simulink model "racing_modes_R2022a"  (R2022a)
settings: Solver=VariableStepAuto  StartTime=0.0  StopTime=10.0  RelTol=1e-3
settings Model: Creator=no  LastModifiedBy=no
settings ModelReferenceCC: EnableRefExpFcnMdlSchedulingChecks=off
settings RTWCC: Description=Generic Real-Time Target

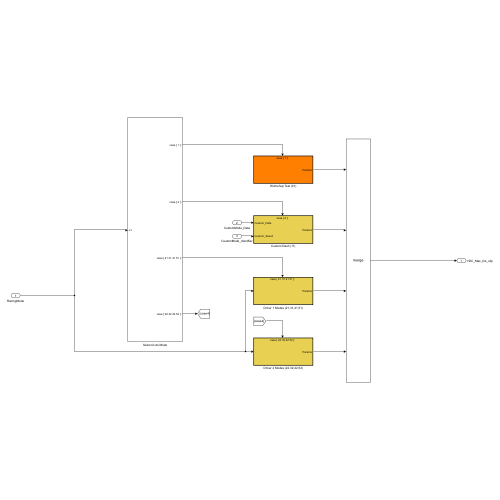
[thumbnail: Simulink's stored preview of the top-level diagram]
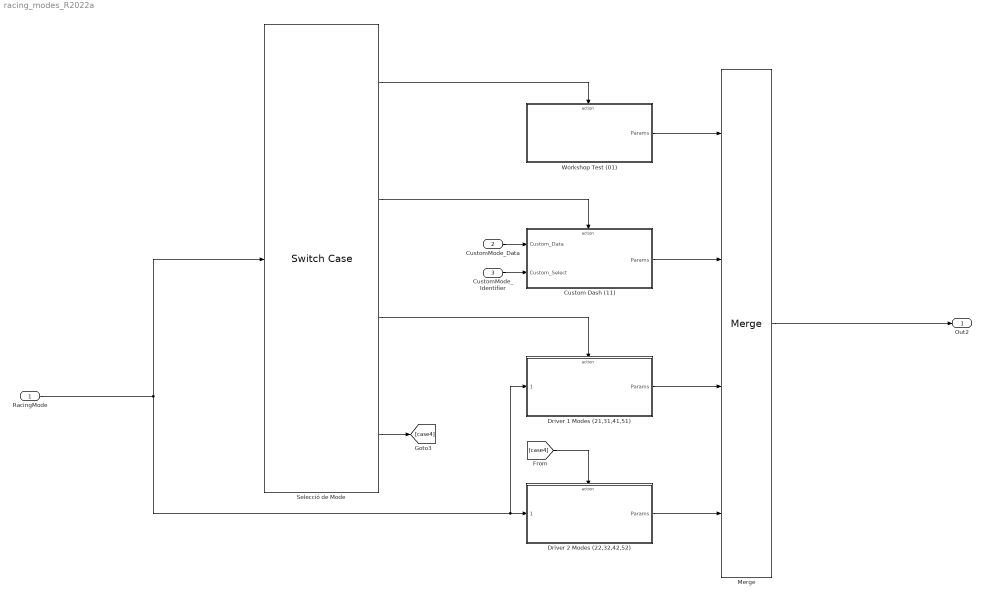
== system racing_modes_R2022a ==
  RacingMode : Inport  OutDataTypeStr=uint8
  CustomMode_Data : Inport  Port=2
  CustomMode_Identifier : Inport  Port=3
  Custom Dash (11) : Subsystem  TreatAsAtomicUnit=on
  Driver 1 Modes (21,31,41,51) : Subsystem  TreatAsAtomicUnit=on
  Driver 2 Modes (22,32,42,52) : Subsystem  TreatAsAtomicUnit=on
  Merge : Merge  Inputs=4
  Selecció de Mode : SwitchCase  CaseConditions={01, 2, [21,31,41,51], [22,32,42,52]}  ShowDefaultCase=off
  Workshop Test (01) : Subsystem  TreatAsAtomicUnit=on
  Out2 : Outport  SignalName=VDC_Max_tire_slip
  wires:
  CustomMode_Identifier/1 -> Custom Dash (11)/2(Custom_Select)
  Custom Dash (11)/1(Params) -> Merge/2
  RacingMode/1 -> Driver 1 Modes (21,31,41,51)/1(" "), Driver 2 Modes (22,32,42,52)/1(" "), Selecció de Mode/1
  Workshop Test (01)/1(Params) -> Merge/1
  CustomMode_Data/1 -> Custom Dash (11)/1(Custom_Data)
  Driver 1 Modes (21,31,41,51)/1(Params) -> Merge/3
  Driver 2 Modes (22,32,42,52)/1(Params) -> Merge/4
  Selecció de Mode/4 -> [case4]
  [case4] -> Driver 2 Modes (22,32,42,52)/Action
  Selecció de Mode/1 -> Workshop Test (01)/Action
  Selecció de Mode/2 -> Custom Dash (11)/Action
  Selecció de Mode/3 -> Driver 1 Modes (21,31,41,51)/Action
  Merge/1 -> Out2/1

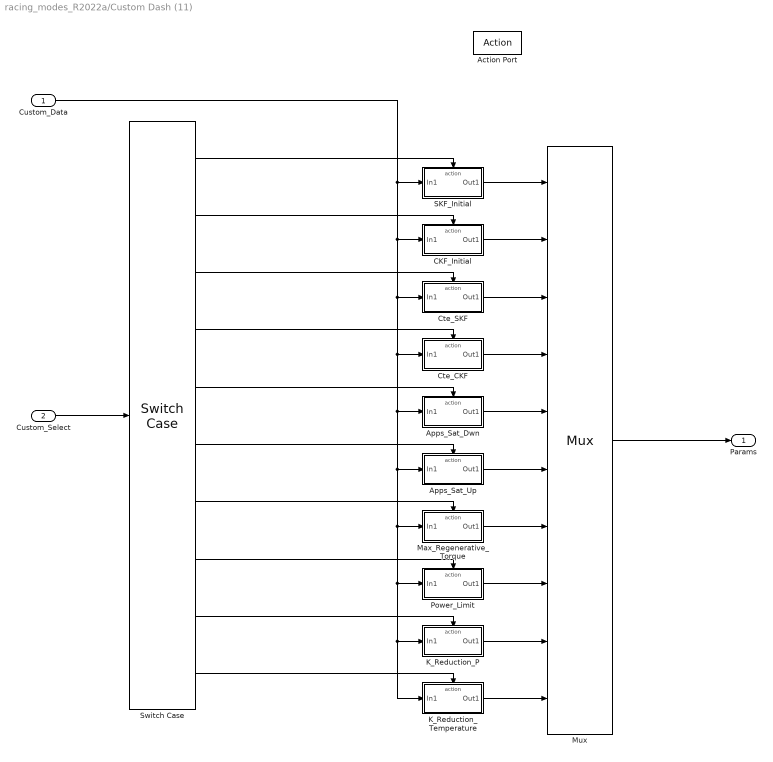
== system racing_modes_R2022a/Custom Dash (11) ==
  Custom_Data : Inport
  Custom_Select : Inport  Port=2
  Action Port : ActionPort  ActionPortLabel=case [ 2 ]:
  Apps_Sat_Dwn : Subsystem  TreatAsAtomicUnit=on
  Apps_Sat_Up : Subsystem  TreatAsAtomicUnit=on
  CKF_Initial : Subsystem  TreatAsAtomicUnit=on
  Cte_CKF : Subsystem  TreatAsAtomicUnit=on
  Cte_SKF : Subsystem  TreatAsAtomicUnit=on
  K_Reduction_P : Subsystem  TreatAsAtomicUnit=on
  K_Reduction_Temperature : Subsystem  TreatAsAtomicUnit=on
  Max_Regenerative_Torque : Subsystem  TreatAsAtomicUnit=on
  Mux : Mux  Inputs=10
  Power_Limit : Subsystem  TreatAsAtomicUnit=on
  SKF_Initial : Subsystem  TreatAsAtomicUnit=on
  Switch Case : SwitchCase  CaseConditions={1,2,3,4,5,6,7,8,9,10}  ShowDefaultCase=off
  Params : Outport  VectorParamsAs1DForOutWhenUnconnected=off
  wires:
  Custom_Select/1 -> Switch Case/1
  Custom_Data/1 -> K_Reduction_Temperature/1(In1), K_Reduction_P/1(In1), Power_Limit/1(In1), Max_Regenerative_Torque/1(In1), Apps_Sat_Up/1(In1), Apps_Sat_Dwn/1(In1), Cte_CKF/1(In1), Cte_SKF/1(In1), CKF_Initial/1(In1), SKF_Initial/1(In1)
  Switch Case/1 -> SKF_Initial/Action
  SKF_Initial/1(Out1) -> Mux/1
  Mux/1 -> Params/1
  CKF_Initial/1(Out1) -> Mux/2
  Cte_SKF/1(Out1) -> Mux/3
  Cte_CKF/1(Out1) -> Mux/4
  Apps_Sat_Dwn/1(Out1) -> Mux/5
  Apps_Sat_Up/1(Out1) -> Mux/6
  Max_Regenerative_Torque/1(Out1) -> Mux/7
  Power_Limit/1(Out1) -> Mux/8
  K_Reduction_P/1(Out1) -> Mux/9
  K_Reduction_Temperature/1(Out1) -> Mux/10
  Switch Case/2 -> CKF_Initial/Action
  Switch Case/3 -> Cte_SKF/Action
  Switch Case/4 -> Cte_CKF/Action
  Switch Case/5 -> Apps_Sat_Dwn/Action
  Switch Case/6 -> Apps_Sat_Up/Action
  Switch Case/7 -> Max_Regenerative_Torque/Action
  Switch Case/8 -> Power_Limit/Action
  Switch Case/9 -> K_Reduction_P/Action
  Switch Case/10 -> K_Reduction_Temperature/Action

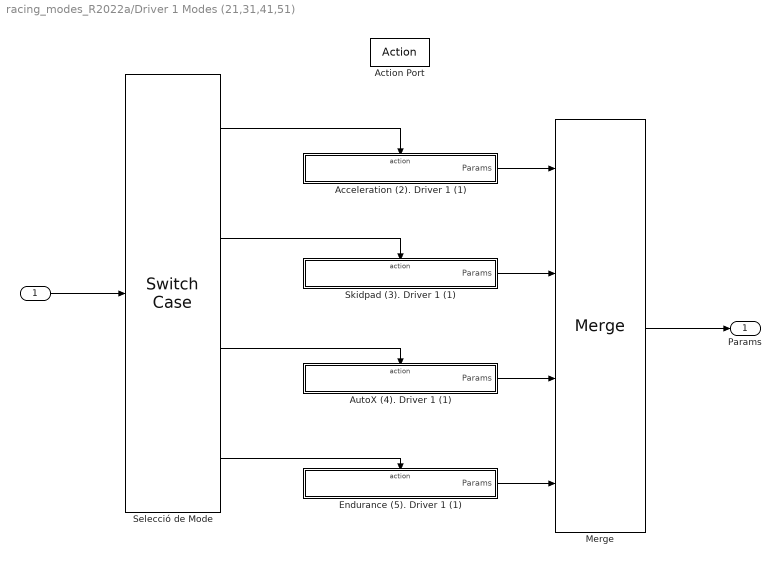
== system racing_modes_R2022a/Driver 1 Modes (21,31,41,51) ==
  " " : Inport  OutDataTypeStr=uint8
  Action Port : ActionPort  ActionPortLabel=case [ 21 31 41 51 ]:
  "Acceleration (2). Driver 1 (1) " : Subsystem  TreatAsAtomicUnit=on
  AutoX (4). Driver 1 (1) : Subsystem  TreatAsAtomicUnit=on
  Endurance (5). Driver 1 (1) : Subsystem  TreatAsAtomicUnit=on
  Merge : Merge  Inputs=4
  Selecció de Mode : SwitchCase  CaseConditions={21,31,41,51}  ShowDefaultCase=off
  Skidpad (3). Driver 1 (1) : Subsystem  TreatAsAtomicUnit=on
  Params : Outport  VectorParamsAs1DForOutWhenUnconnected=off
  wires:
  Merge/1 -> Params/1
  " "/1 -> Selecció de Mode/1
  Selecció de Mode/4 -> Endurance (5). Driver 1 (1)/Action
  Selecció de Mode/3 -> AutoX (4). Driver 1 (1)/Action
  Selecció de Mode/2 -> Skidpad (3). Driver 1 (1)/Action
  Selecció de Mode/1 -> "Acceleration (2). Driver 1 (1) "/Action
  "Acceleration (2). Driver 1 (1) "/1(Params) -> Merge/1
  Skidpad (3). Driver 1 (1)/1(Params) -> Merge/2
  AutoX (4). Driver 1 (1)/1(Params) -> Merge/3
  Endurance (5). Driver 1 (1)/1(Params) -> Merge/4

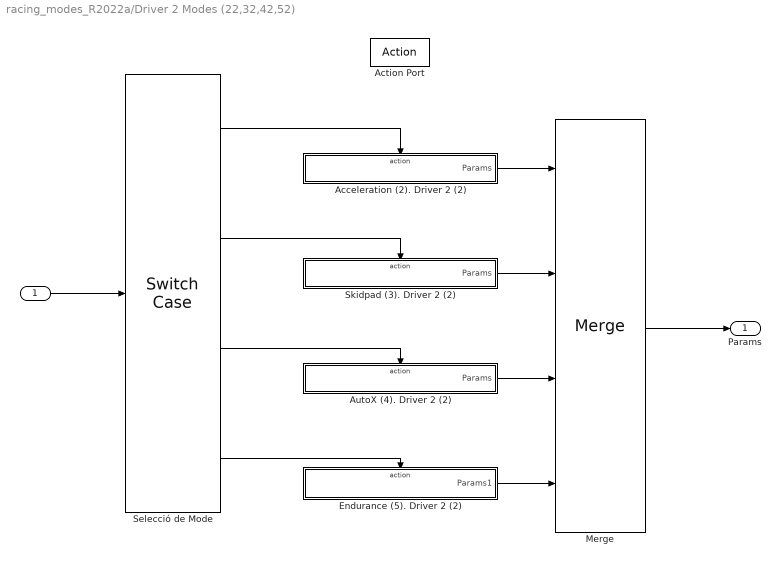
== system racing_modes_R2022a/Driver 2 Modes (22,32,42,52) ==
  " " : Inport  OutDataTypeStr=uint8
  Action Port : ActionPort  ActionPortLabel=case [ 22 32 42 52 ]:
  "Acceleration (2). Driver 2 (2) " : Subsystem  TreatAsAtomicUnit=on
  AutoX (4). Driver 2 (2) : Subsystem  TreatAsAtomicUnit=on
  Endurance (5). Driver 2 (2) : Subsystem  TreatAsAtomicUnit=on
  Merge : Merge  Inputs=4
  Selecció de Mode : SwitchCase  CaseConditions={22,32,42,52}  ShowDefaultCase=off
  Skidpad (3). Driver 2 (2) : Subsystem  TreatAsAtomicUnit=on
  Params : Outport  VectorParamsAs1DForOutWhenUnconnected=off
  wires:
  Merge/1 -> Params/1
  " "/1 -> Selecció de Mode/1
  Selecció de Mode/4 -> Endurance (5). Driver 2 (2)/Action
  Selecció de Mode/3 -> AutoX (4). Driver 2 (2)/Action
  Selecció de Mode/2 -> Skidpad (3). Driver 2 (2)/Action
  Selecció de Mode/1 -> "Acceleration (2). Driver 2 (2) "/Action
  "Acceleration (2). Driver 2 (2) "/1(Params) -> Merge/1
  Skidpad (3). Driver 2 (2)/1(Params) -> Merge/2
  AutoX (4). Driver 2 (2)/1(Params) -> Merge/3
  Endurance (5). Driver 2 (2)/1(Params1) -> Merge/4

== system racing_modes_R2022a/Workshop Test (01) ==
  Action Port : ActionPort  ActionPortLabel=case [ 1 ]:
  Max tyre slip : Constant
  Params : Outport  VectorParamsAs1DForOutWhenUnconnected=off
  wires:
  Max tyre slip/1 -> Params/1

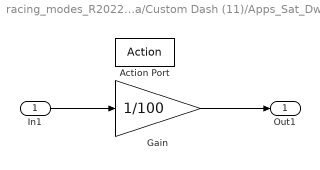
== system racing_modes_R2022a/Custom Dash (11)/Apps_Sat_Dwn ==
  In1 : Inport
  Action Port : ActionPort
  Gain : Gain  Gain=1/100
  Out1 : Outport  VectorParamsAs1DForOutWhenUnconnected=off
  wires:
  In1/1 -> Gain/1
  Gain/1 -> Out1/1

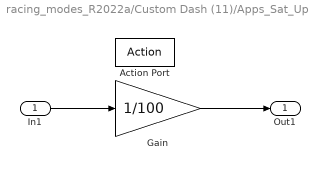
== system racing_modes_R2022a/Custom Dash (11)/Apps_Sat_Up ==
  In1 : Inport
  Action Port : ActionPort
  Gain : Gain  Gain=1/100
  Out1 : Outport  VectorParamsAs1DForOutWhenUnconnected=off
  wires:
  In1/1 -> Gain/1
  Gain/1 -> Out1/1

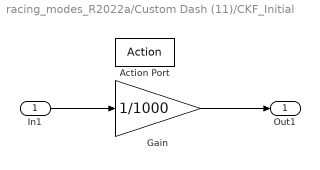
== system racing_modes_R2022a/Custom Dash (11)/CKF_Initial ==
  In1 : Inport
  Action Port : ActionPort
  Gain : Gain  Gain=1/1000
  Out1 : Outport  VectorParamsAs1DForOutWhenUnconnected=off
  wires:
  In1/1 -> Gain/1
  Gain/1 -> Out1/1

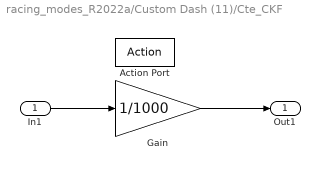
== system racing_modes_R2022a/Custom Dash (11)/Cte_CKF ==
  In1 : Inport
  Action Port : ActionPort
  Gain : Gain  Gain=1/1000
  Out1 : Outport  VectorParamsAs1DForOutWhenUnconnected=off
  wires:
  In1/1 -> Gain/1
  Gain/1 -> Out1/1

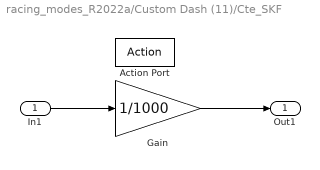
== system racing_modes_R2022a/Custom Dash (11)/Cte_SKF ==
  In1 : Inport
  Action Port : ActionPort
  Gain : Gain  Gain=1/1000
  Out1 : Outport  VectorParamsAs1DForOutWhenUnconnected=off
  wires:
  In1/1 -> Gain/1
  Gain/1 -> Out1/1

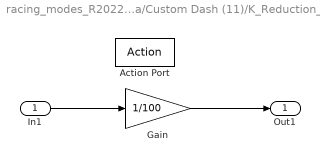
== system racing_modes_R2022a/Custom Dash (11)/K_Reduction_P ==
  In1 : Inport
  Action Port : ActionPort
  Gain : Gain  Gain=1/100
  Out1 : Outport  VectorParamsAs1DForOutWhenUnconnected=off
  wires:
  In1/1 -> Gain/1
  Gain/1 -> Out1/1

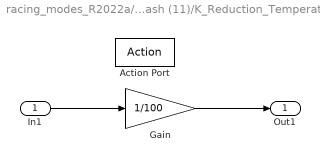
== system racing_modes_R2022a/Custom Dash (11)/K_Reduction_Temperature ==
  In1 : Inport
  Action Port : ActionPort
  Gain : Gain  Gain=1/100
  Out1 : Outport  VectorParamsAs1DForOutWhenUnconnected=off
  wires:
  In1/1 -> Gain/1
  Gain/1 -> Out1/1

== system racing_modes_R2022a/Custom Dash (11)/Max_Regenerative_Torque ==
  In1 : Inport
  Action Port : ActionPort
  Out1 : Outport  VectorParamsAs1DForOutWhenUnconnected=off
  wires:
  In1/1 -> Out1/1

== system racing_modes_R2022a/Custom Dash (11)/Power_Limit ==
  In1 : Inport
  Action Port : ActionPort
  Out1 : Outport  VectorParamsAs1DForOutWhenUnconnected=off
  wires:
  In1/1 -> Out1/1

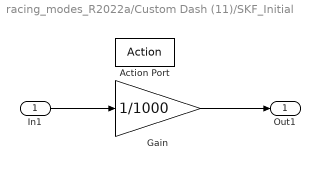
== system racing_modes_R2022a/Custom Dash (11)/SKF_Initial ==
  In1 : Inport
  Action Port : ActionPort
  Gain : Gain  Gain=1/1000
  Out1 : Outport  VectorParamsAs1DForOutWhenUnconnected=off
  wires:
  In1/1 -> Gain/1
  Gain/1 -> Out1/1

== system racing_modes_R2022a/Driver 1 Modes (21,31,41,51)/Acceleration (2). Driver 1 (1)  ==
  Action Port : ActionPort
  Max tyre slip : Constant
  Params : Outport  VectorParamsAs1DForOutWhenUnconnected=off
  wires:
  Max tyre slip/1 -> Params/1

== system racing_modes_R2022a/Driver 1 Modes (21,31,41,51)/AutoX (4). Driver 1 (1) ==
  Action Port : ActionPort
  Max tyre slip : Constant
  Params : Outport  VectorParamsAs1DForOutWhenUnconnected=off
  wires:
  Max tyre slip/1 -> Params/1

== system racing_modes_R2022a/Driver 1 Modes (21,31,41,51)/Endurance (5). Driver 1 (1) ==
  Action Port : ActionPort
  Max tyre slip : Constant
  Params : Outport  VectorParamsAs1DForOutWhenUnconnected=off
  wires:
  Max tyre slip/1 -> Params/1

== system racing_modes_R2022a/Driver 1 Modes (21,31,41,51)/Skidpad (3). Driver 1 (1) ==
  Action Port : ActionPort
  Max tyre slip : Constant
  Params : Outport  VectorParamsAs1DForOutWhenUnconnected=off
  wires:
  Max tyre slip/1 -> Params/1

== system racing_modes_R2022a/Driver 2 Modes (22,32,42,52)/Acceleration (2). Driver 2 (2)  ==
  Action Port : ActionPort
  Max tyre slip : Constant
  Params : Outport  VectorParamsAs1DForOutWhenUnconnected=off
  wires:
  Max tyre slip/1 -> Params/1

== system racing_modes_R2022a/Driver 2 Modes (22,32,42,52)/AutoX (4). Driver 2 (2) ==
  Action Port : ActionPort
  Max tyre slip : Constant
  Params : Outport  VectorParamsAs1DForOutWhenUnconnected=off
  wires:
  Max tyre slip/1 -> Params/1

== system racing_modes_R2022a/Driver 2 Modes (22,32,42,52)/Endurance (5). Driver 2 (2) ==
  Action Port : ActionPort
  Max tyre slip1 : Constant
  Params1 : Outport  VectorParamsAs1DForOutWhenUnconnected=off
  wires:
  Max tyre slip1/1 -> Params1/1

== system racing_modes_R2022a/Driver 2 Modes (22,32,42,52)/Skidpad (3). Driver 2 (2) ==
  Action Port : ActionPort
  Max tyre slip : Constant
  Params : Outport  VectorParamsAs1DForOutWhenUnconnected=off
  wires:
  Max tyre slip/1 -> Params/1
